simulink model "Task_6"  (R2020b)
settings: Solver=FixedStepDiscrete  StartTime=0.0  StopTime=10.0  RelTol=1e-3
settings Model: Creator=hp  LastModifiedBy=hp
settings OptimizationCC: DefaultParameterBehavior=Inlined  EnhancedBackFolding=on  PassReuseOutputArgsAs=Individual arguments  ZeroExternalMemoryAtStartup=off  ZeroInternalMemoryAtStartup=off  OptimizeBlockOrder=speed  DifferentSizesBufferReuse=on  OptimizationCustomize=off  EfficientTunableParamExpr=on
settings DebuggingCC: UnderspecifiedInitializationDetection=Classic  MergeDetectMultiDrivingBlocksExec=none  ParameterTunabilityLossMsg=error
settings ModelReferenceCC: PropagateSignalLabelsOutOfModel=off
settings SFSimCC: MATLABDynamicMemAlloc=off
settings RTWCC: Description=Create Visual C/C++ Solution File for Embedded Coder  SystemTargetFile=ert.tlc  GenCodeOnly=on  TemplateMakefile=RTW.MSVCBuild  GenerateReport=on  IncludeHyperlinkInReport=on  LaunchReport=on  GenerateTraceInfo=on  GenerateTraceReport=on  GenerateTraceReportSl=on  GenerateTraceReportSf=on  GenerateTraceReportEml=on  GenerateCodeReplacementReport=on
settings CodeAppCC: ForceParamTrailComments=on  IgnoreCustomStorageClasses=off  OperatorAnnotations=on  SimulinkDataObjDesc=on  SFDataObjDesc=on  InsertBlockDesc=on
settings ERTTargetCC: TargetLangStandard=C99 (ISO)  GenerateSampleERTMain=on  InlinedParameterPlacement=NonHierarchical  ERTCustomFileTemplate=example_file_process.tlc

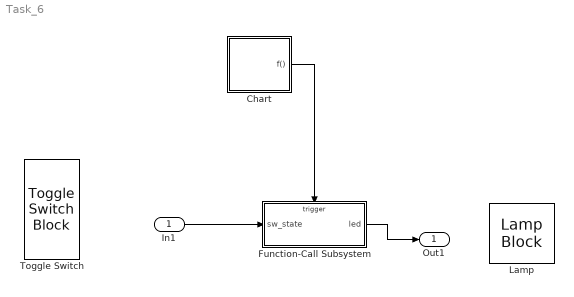
== system Task_6 ==
  In1 : Inport
  Chart : Stateflow chart  TreatAsAtomicUnit=on
  Function-Call Subsystem : Subsystem  TreatAsAtomicUnit=on
  Lamp : LampBlock
  Toggle Switch : ToggleSwitchBlock
      settings: Values={{'Off', 'On'}, [0 1]}
  Out1 : Outport
  wires:
  In1/1 -> Function-Call Subsystem/1(sw_state)
  Function-Call Subsystem/1(led) -> Out1/1
  Chart/1(f()) -> Function-Call Subsystem/Trigger

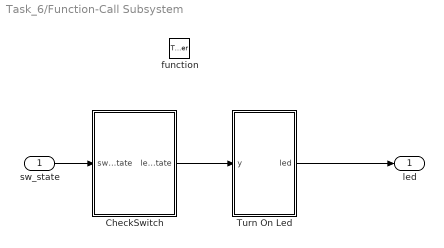
== system Task_6/Function-Call Subsystem ==
  sw_state : Inport
  function : TriggerPort  TriggerType=function-call  VariantControl=Variant
  CheckSwitch : Stateflow chart  TreatAsAtomicUnit=on
  Turn On Led : Stateflow chart  TreatAsAtomicUnit=on
  led : Outport
  wires:
  sw_state/1 -> CheckSwitch/1(sw_state)
  CheckSwitch/1(ledstate) -> Turn On Led/1(y)
  Turn On Led/1(led) -> led/1

== stateflow chart Task_6/Function-Call Subsystem/CheckSwitch ==
  (default) -> (junction 7) : % check switch
  (junction 7) -> (junction 8) [order 1] : [sw_state==1]
  (junction 7) -> (junction 9) [order 2] : {ledstate=0;}
  (junction 8) -> (junction 10) : {ledstate=1;}
  (junction 10) -> (junction 9)
  (junction 9) -> (junction 11)
  data: sw_state input; ledstate output

== stateflow chart Task_6/Function-Call Subsystem/Turn On Led ==
  (default) -> (junction 7) : % ledStatus
  (junction 7) -> (junction 8) [order 1] : [y == 1]
  (junction 7) -> (junction 9) [order 2] : {led=0;}
  (junction 8) -> (junction 10) : {led=1;}
  (junction 10) -> (junction 9)
  (junction 9) -> (junction 11)
  data: y input; led output

== stateflow chart Task_6/Chart ==
  state state1
    en:
    du:
    ex:
  (default) -> state1
  state1 -> state1 : [after(5,tick)]{f;}
  events: f output FUNCTION_CALL_EVENT
